simulink model "ask_modulation"  (R2025a)
settings: Solver=VariableStepAuto  StartTime=0.0  StopTime=10.0  RelTol=1e-3
libraries: commchan3 x1, commrandsrc3 x1, commsink2 x1
settings Model: Creator=Bremdow  LastModifiedBy=Bremdow

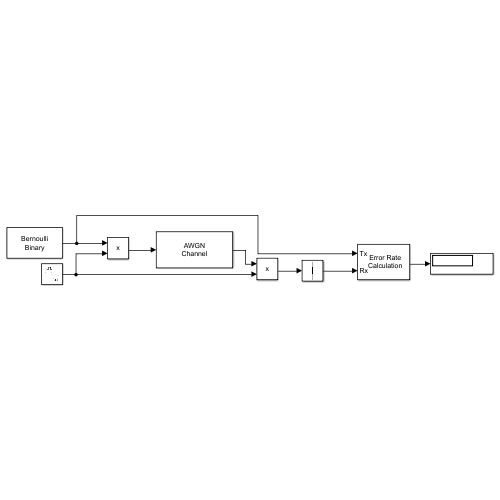
[thumbnail: Simulink's stored preview of the top-level diagram]
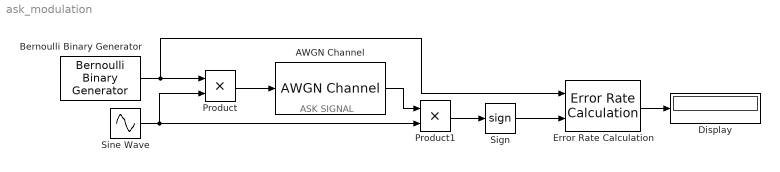
== system ask_modulation ==
  note: ASK SIGNAL
  AWGN Channel : commchan3/AWGN Channel  LegacyMode=off  NoiseMethod="Signal to noise ratio  (SNR)"  noiseMode="Signal to noise ratio  (SNR)"  EbNo=10  EsNo=10  SNR=10  BitsPerSymbol=1  SignalPower=1  SpecifySymbolPeriod=off  SamplesPerSymbol=1  SymbolPeriod=1  VarianceSource=Parameter  Variance=1  RandomStream=Global stream  Seed=67  SimulateUsing=Code generation
  Bernoulli Binary Generator : commrandsrc3/Bernoulli Binary Generator  ProbabilityOfZero=0.5  SeedSource=Auto  Seed=0  SampleTime=61  SamplesPerFrame=1  OutputDataType=double  SimulateUsing=Interpreted execution
  Display : Display
  Error Rate Calculation : commsink2/Error Rate Calculation  N=0  st_delay=0  cp_mode=Entire frame  subframe=[]  PMode=Port  WsName=ErrorVec  RsMode2=off  stop=off  numErr=100  maxBits=1e6
      settings: LibrarySourceBlock=|
      | commhdlsink/Error Rate
      | Calculation
  Product : Product
  Product1 : Product
  Sign : Signum
  Sine Wave : Sin  Frequency=2*pi*10  SampleTime=0.01
  wires:
  Sine Wave/1 -> Product1/2, Product/2
  Bernoulli Binary Generator/1 -> Error Rate Calculation/1, Product/1
  Product/1 -> AWGN Channel/1
  AWGN Channel/1 -> Product1/1
  Product1/1 -> Sign/1
  Sign/1 -> Error Rate Calculation/2
  Error Rate Calculation/1 -> Display/1
